simulink model "half_code_trim"  (R2014a)
settings: Solver=ode45  StartTime=0.0  StopTime=500.0  RelTol=1e-3
values from neighbouring files (symbols this model uses):
  Ixx = 1285.31    [init_coeff_Cessna.m]
  Ixy = 0.0    (= 0)    [init_coeff_Cessna.m]
  Ixz = 0.0    (= 0)    [init_coeff_Cessna.m]
  Iyx = Ixy    (= 0)    [init_coeff_Cessna.m]
  Iyy = 1824.93    [init_coeff_Cessna.m]
  Iyz = 0.0    (= 0)    [init_coeff_Cessna.m]
  Izx = Ixz    (= 0)    [init_coeff_Cessna.m]
  Izy = Iyz    (= 0)    [init_coeff_Cessna.m]
  Izz = 2666.893    [init_coeff_Cessna.m]
  p_init = 0    [trim_simulate.m]
  phi_init = 0    [trim_simulate.m]
  psi_init = 0    [trim_simulate.m]
  q_init = 0    [trim_simulate.m]
  r_init = 0    [trim_simulate.m]
  theta_init = 0.0105    [trim_simulate.m]
  u_init = 80.00    (= 80)    [trim_simulate.m]
  v_init = 0.00    (= 0)    [trim_simulate.m]
  w_init = 0    [trim_simulate.m]
  xe_init = 0    [trim_simulate.m]
  ye_init = 0    [trim_simulate.m]
  ze_init = -200    [trim_simulate.m]
libraries: aerolibobsolete x1, aerolibasang x1
settings Model: Creator=sajith  LastModifiedBy=sajith
settings DataIOCC: SignalLoggingSaveFormat=ModelDataLogs
settings OptimizationCC: ExpressionDepthLimit=2147483647
settings DebuggingCC: UnderspecifiedInitializationDetection=Classic  FcnCallInpInsideContextMsg=UseLocalSettings  StateNameClashWarn=warning
settings SFSimCC: SimParseCustomCode=off
settings GRTTargetCC: CombineOutputUpdateFcns=off  GRTInterface=on

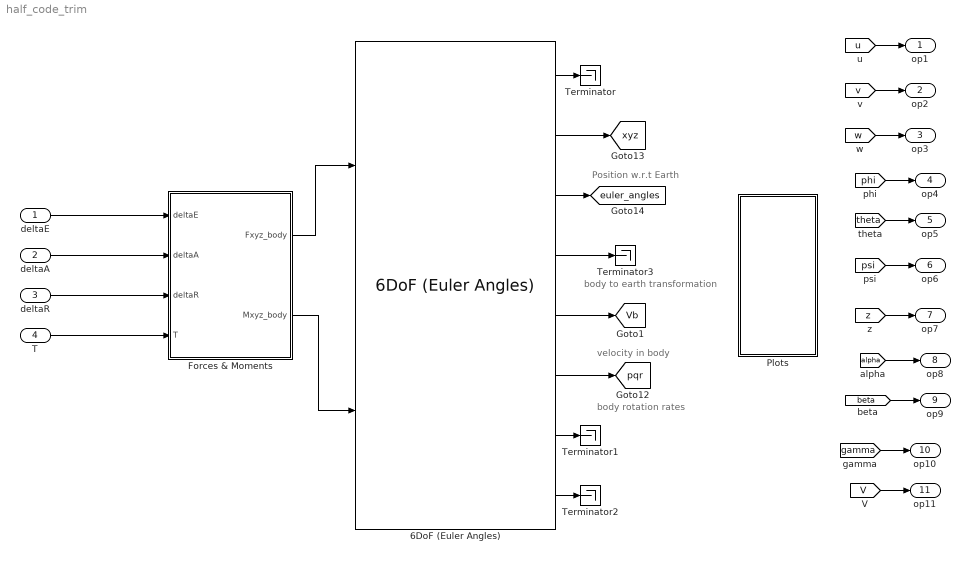
== system half_code_trim ==
  note: velocity in body
  note: body rotation rates
  note: body to earth transformation
  note: Position w.r.t Earth
  deltaE : Inport
  deltaA : Inport  Port=2
  deltaR : Inport  Port=3
  T : Inport  Port=4
  6DoF (Euler Angles) : aerolibobsolete/6DoF (Euler Angles)  units=Metric (MKS)  mtype=Fixed  rep=Euler Angles  xme_0=[xe_init ye_init ze_init]  Vm_0=[u_init v_init w_init]  eul_0=[phi_init theta_init psi_init]  pm_0=[p_init q_init r_init]  mass_0=mass  mass_e=0.5  mass_f=2.0  inertia=[Ixx Ixy Ixz;Iyx Iyy Iyz;Izx Izy Izz]  inertia_e=eye(3)  inertia_f=2*eye(3)  k_quat=1.0
  Forces & Moments : Subsystem
  Plots : Subsystem
  Terminator{,1..3} (4 alike) : Terminator
  op1 : Outport
  op2 : Outport  Port=2
  op3 : Outport  Port=3
  op4 : Outport  Port=4
  op5 : Outport  Port=5
  op6 : Outport  Port=6
  op7 : Outport  Port=7
  op8 : Outport  Port=8
  op9 : Outport  Port=9
  op10 : Outport  Port=10
  op11 : Outport  Port=11
  tag scope: Vb=global, euler_angles=global, pqr=global, xyz=global
  wires:
  deltaE/1 -> Forces & Moments/1(deltaE)
  deltaA/1 -> Forces & Moments/2(deltaA)
  deltaR/1 -> Forces & Moments/3(deltaR)
  T/1 -> Forces & Moments/4(T)
  [u] -> op1/1
  [v] -> op2/1
  [w] -> op3/1
  [phi] -> op4/1
  [theta] -> op5/1
  [psi] -> op6/1
  [z] -> op7/1
  [alpha] -> op8/1
  [beta] -> op9/1
  [gamma] -> op10/1
  [V] -> op11/1
  Forces & Moments/1(Fxyz_body) -> 6DoF (Euler Angles)/1
  Forces & Moments/2(Mxyz_body) -> 6DoF (Euler Angles)/2
  6DoF (Euler Angles)/2 -> [xyz]
  6DoF (Euler Angles)/3 -> [euler_angles]
  6DoF (Euler Angles)/4 -> Terminator3/1
  6DoF (Euler Angles)/6 -> [pqr]
  6DoF (Euler Angles)/5 -> [Vb]
  6DoF (Euler Angles)/1 -> Terminator/1
  6DoF (Euler Angles)/7 -> Terminator1/1
  6DoF (Euler Angles)/8 -> Terminator2/1

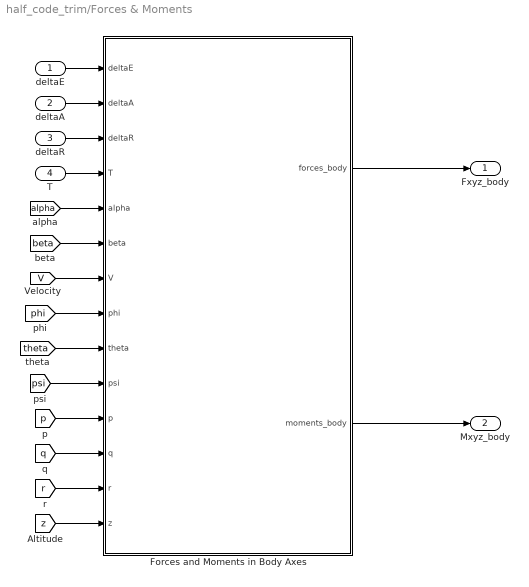
== system half_code_trim/Forces & Moments ==
  deltaE : Inport
  deltaA : Inport  Port=2
  deltaR : Inport  Port=3
  T : Inport  Port=4
  Forces and Moments in Body Axes : MATLAB Function  TreatAsAtomicUnit=on
  Fxyz_body : Outport
  Mxyz_body : Outport  Port=2
  wires:
  Forces and Moments in Body Axes/1(forces_body) -> Fxyz_body/1
  Forces and Moments in Body Axes/2(moments_body) -> Mxyz_body/1
  [alpha] -> Forces and Moments in Body Axes/5(alpha)
  [beta] -> Forces and Moments in Body Axes/6(beta)
  [V] -> Forces and Moments in Body Axes/7(V)
  [phi] -> Forces and Moments in Body Axes/8(phi)
  [theta] -> Forces and Moments in Body Axes/9(theta)
  [psi] -> Forces and Moments in Body Axes/10(psi)
  [p] -> Forces and Moments in Body Axes/11(p)
  [q] -> Forces and Moments in Body Axes/12(q)
  [r] -> Forces and Moments in Body Axes/13(r)
  deltaE/1 -> Forces and Moments in Body Axes/1(deltaE)
  T/1 -> Forces and Moments in Body Axes/4(T)
  deltaA/1 -> Forces and Moments in Body Axes/2(deltaA)
  deltaR/1 -> Forces and Moments in Body Axes/3(deltaR)
  [z] -> Forces and Moments in Body Axes/14(z)

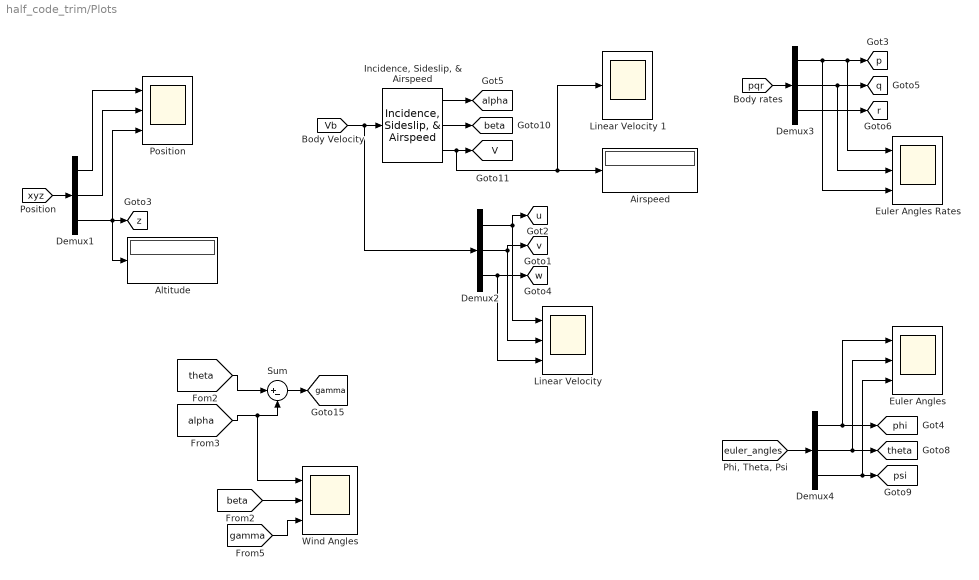
== system half_code_trim/Plots ==
  Airspeed : Display
  Altitude : Display
  Demux{1..4} (4 alike) : Demux  Outputs=3
  Euler Angles : Scope  NumInputPorts=3
      settings: YMin=-5~-5~-5  YMax=5~5~5  SaveName=ScopeData2
  Euler Angles Rates : Scope  NumInputPorts=3
      settings: YMin=-5~-5~-5  YMax=5~5~5  SaveName=ScopeData3
  "Incidence, Sideslip, & Airspeed" : aerolibasang/Incidence, Sideslip, & Airspeed
  "Linear Velocity " : Scope  NumInputPorts=3
      settings: YMin=-5~-5~-5  YMax=5~5~5  SaveName=ScopeData4
  Linear Velocity 1 : Scope
      settings: SaveName=ScopeData5
  Position : Scope  NumInputPorts=3
      settings: YMin=-5~-5~-5  YMax=5~5~5
  Sum : Sum  Inputs=|+-
  Wind Angles : Scope  NumInputPorts=3
      settings: YMin=-5~-5~-5  YMax=5~5~5
  tag scope: V=global, alpha=global, beta=global, gamma=global, p=global, phi=global, psi=global, q=global, r=global, theta=global, u=global, v=global, w=global, z=global
  wires:
  Demux1/1 -> Position/1
  Demux1/2 -> Position/2
  Demux1/3 -> Altitude/1, [z], Position/3
  Demux2/3 -> [w], "Linear Velocity "/3
  Demux2/2 -> [v], "Linear Velocity "/2
  Demux2/1 -> [u], "Linear Velocity "/1
  Demux3/3 -> [r]
  Demux3/2 -> [q], Euler Angles Rates/2
  Demux3/1 -> [p], Euler Angles Rates/1, Euler Angles Rates/3
  Demux4/3 -> [psi], Euler Angles/3
  Demux4/2 -> [theta], Euler Angles/2
  Demux4/1 -> [phi], Euler Angles/1
  "Incidence, Sideslip, & Airspeed"/1 -> [alpha]
  "Incidence, Sideslip, & Airspeed"/2 -> [beta]
  "Incidence, Sideslip, & Airspeed"/3 -> [V], Linear Velocity 1/1, Airspeed/1
  [theta] -> Sum/1
  [alpha] -> Sum/2, Wind Angles/1
  Sum/1 -> [gamma]
  [beta] -> Wind Angles/2
  [gamma] -> Wind Angles/3
  [xyz] -> Demux1/1
  [euler_angles] -> Demux4/1
  [Vb] -> Demux2/1, "Incidence, Sideslip, & Airspeed"/1
  [pqr] -> Demux3/1

== matlab function half_code_trim/Forces & Moments/Forces and Moments in Body Axes ==
  data: deltaE input; forces_body output; deltaA input; deltaR input; T input; alpha input; beta input; V input; phi input; theta input; psi input; p input; q input; r input; moments_body output; z input
function [forces_body,moments_body] = fcn(deltaE,deltaA,deltaR,T,alpha,beta,V,phi,theta,psi,p,q,r,z)
%#codegen

%% environmental constants
g = 9.8; % acceleration due to gravity


%% geometric quantities
c_bar=1.493; % chord length
b=10.911; % wing span
S=16.1651; % wing area

%% mass and inertia
mass = 1043.26; % mass
Ixx=1285.31;
Ixy=0.0;
Iyx=Ixy;
Ixz=0.0;
Izx=Ixz;
Iyy= 1824.93; % moment of inertia
Iyz=0.0;
Izy=Iyz;
Izz=2666.893;

%% aerodynamic coefficients
% drag
cd0=0.036;
cd_alpha = 0.13;
k_drag=0.0830304;
cd_delta_e=0.06;
cd_beta=0.17;

%side force
cy_beta=-0.31;
cy_p=-0.037;
cy_r=0.21;
cy_delta_r=0.187;
cy_delta_a=0;

% lift
cl0=0.25;
cl_alpha=4.47;
cl_q=3.9;
cl_delta_e=0.3476;

% rolling moment
c_l_beta=-0.089;
c_l_p=-0.47;
c_l_r=0.096;
c_l_delta_a=-0.09;
c_l_delta_r=0.0147;

% pitching moment
cm0=-0.02;
cm_alpha=-1.8;
cm_alpha_dot=0.0;
cm_q=-12.4;
cm_delta_e=-1.28;
alpha_dot=0;

% yawing moment
cn_beta=0.065;
cn_p=-0.03;
cn_r=-0.99;
cn_delta_a=-0.0053;
cn_delta_r=-0.0657;



%% Calculations

%%%%%%% Calculation of density with respect to altitude
R = 287;
h = -z;  % z direction is downwards

if (h <= 11000)  % temperature gradient region
    Temp = 288.16 - 6.5*10^(-3)*h;
    rho = 1.225 * (Temp/288.16)^(-((g/(-6.5*10^(-3)*R))+1));
    
    
elseif (h > 11000 && h <= 25000) % isothermal region
    rho = 0.3639 * exp(-(g/(R*216.66))*(h-11000));
    

elseif (h > 25000 && h <= 45000) % temperature gradient region
    Temp = 216.66 + 3*10^(-3)*(h-25000);
    rho = 0.03946 * (Temp/216.66)^(-1*((g/(0.003*R))+1));
else 
    rho = 0.08;

end


W = mass*g; %weight

qd = 0.5*rho*V^2; % Dynamic pressure


p_cap = p*b/(2*V);
q_cap = q*c_bar/(2*V);
r_cap = r*b/(2*V);




C_L = cl0+cl_alpha*alpha+cl_q*q_cap+cl_delta_e*deltaE; %coef. of lift
%C_D = cd0+cd_alpha*abs(alpha)+cd_beta*abs(beta)+cd_delta_e*abs(deltaE); % coeff. of drag
C_D = cd0 + k_drag*C_L^2;
C_Y = cy_beta*beta+cy_p*p_cap+cy_r*r_cap+cy_delta_a*deltaA; % coeff. of side slip

% coeff. of moments
C_l = c_l_beta*beta+c_l_p*p_cap+c_l_r*r_cap+c_l_delta_a*deltaA+c_l_delta_r*deltaR; % coeff. of moment about X-axis(tendency to roll)
C_m = cm0 +cm_alpha*alpha+cm_alpha_dot*alpha_dot+cm_delta_e*deltaE; % coeff. of moment about Y-axis(tendency to pitch)
C_n = cn_beta*beta+cn_p*p_cap+cn_r*r_cap+cn_delta_a*deltaA+cn_delta_r*deltaR; % coeff. of moment about Z-axis(tendency to yaw)


%forces
L = qd*S*C_L;
D = qd*S*C_D;
Y = qd*S*C_Y;
W = g*mass;

%moments
l = qd*S*C_l*b;
m = qd*S*C_m*c_bar;
n = qd*S*C_n*b;

%transorm to body axes
trans_wind_body = [cos(alpha)*cos(beta)   -cos(alpha)*sin(beta)   -sin(alpha); ...
    sin(beta)                cos(beta)            0     ; ...
    sin(alpha)*cos(beta)   -sin(alpha)*sin(beta)   cos(alpha)];

forces_body = trans_wind_body*[-D Y -L]' + W*[-sin(theta) sin(phi)*cos(theta) cos(phi)*cos(theta)]' + T*[1 0  0]';

moments_body = [l m n]';
